simulink model "MTDC_MODEL"  (R2021a)
settings: Solver=ode1  StartTime=0.0  StopTime=3  FixedStep=2e-5  MaxStep=1e-5  RelTol=1e-5  EnableMultiTasking=on
InitFcn:
  | tau_iac=ts_G_iac/4;                                         %Current loop speed
  | wAC=1/tau_iac;                                              %Frequency
  | L1AC=wAC/s;                                                 %Open loop IMC (L) transfer function to obtain a first order after closing the loop
  | Kp_AC=wAC*(Lg_1+La_1/2);                                    %Proportional constant of the controller
  | Ki_AC=wAC*(Rg_1+Ra_1/2);                                    %Integral constant of the controller
  | C_IMC_AC=(Kp_AC*s+Ki_AC)/s;                                 %IMC designed PI controller transfer function
  | TAC=minreal((C_IMC_AC)*G_iac/(1+(C_IMC_AC)*G_iac));         %Closed loop transfer function
  | 
  | tau_Pac=ts_G_P/4;
  | D = TAC*U_ll1;
  | [C_pi,info] = pidtune(D,'PI',1/tau_Pac);
  | Ki_P = C_pi.Ki;
  | 
  | tau_Qac=ts_G_Q/4;
  | [C_piq,info] = pidtune(D,'PI',1/tau_Qac);
  | Ki_Q = C_piq.Ki;
  | 
  | 
  | tau_isum=ts_G_isum/4;                                        %Current loop speed
  | wsum=1/tau_isum;                                             %Frequency
  | L1AC=wsum/s;                                                 %Open loop IMC (L) transfer function to obtain a first order after closing the loop
  | Kp_sum=wsum*(2*La_1);                                        %Proportional constant of the controller
  | Ki_sum=wsum*(2*Ra_1);                                        %Integral constant of the controller
  | C_IMC_sum=(Kp_sum*s+Ki_sum)/s;                               %IMC designed PI controller transfer function
  | 
  | Kp_sum_PR = wc*(2*La_1);
  | Ki_sum_PR = wc*(2*Ra_1);
  | PR = (Kp_sum_PR*s^2 + 2*wc*(Kp_sum_PR+Ki_sum_PR)*s +Kp_sum_PR*w0^2)/(s^2+2*wc*s+w0^2);
  | 
  | 
  | %Energy reference for a converter arm (sum of all the submodule energies)
  | ArmEnergyRef=1/2*Carm*ArmVoltageRef^2;                      %Energy reference for a converter leg
  | LegEnergy=ArmEnergyRef*2;                                   %References for the controllers (DC side)
  | TotalEnergyRef=ArmEnergyRef*6;                              %Reference of the total energy of the converter
  | EnergyDiffabRef=0;                                          %Reference for the energy difference between legs a and b
  | EnergyDiffacRef=0;                                          %Reference for the energy difference between legs b and c
  | 
  | %References for the controllers (AC side)
  | EnergyDiffUpLowRefa=0;                                      %Reference for the energy difference upper and lower arms of phase a
  | EnergyDiffUpLowRefb=0;                                      %Reference for the energy difference upper and lower arms of phase b
  | EnergyDiffUpLowRefc=0;                                      %Reference for the energy difference upper and lower arms of phase c
  |                                                             %Controller design
  | Kpenergy=50;                                                %Proportional gain
  | Kienergy=20;                                                %Integral gain
  | 
  | Kpenergyt=50;                                               %Proportional gain
  | Kienergyt=20;                                               %Integral gain
  | 
  | Q=3;
  | wn=50*2*pi;                                                 %Frequency to eliminate 50 Hz
  | N_50 = tf([1 0 wn^2],[1 2*wn/Q wn^2]);                       %Notch filter 1 design
  | wn=100*2*pi;                                                %Frequency to eliminate 100 Hz
  | N_100 = tf([1 0 wn^2],[1 2*wn/Q wn^2]);                      %Notch filter 2 design
  | Notch=N_50*N_100;                                            %Combination of both notch filters
  | 
  | Ibasedc1= 1000e6/640e3;                 %Nominal current peak DC
  | IsaturationinnerDC1=1.1*Ibasedc1/3;  %Saturation of the DC inner current
  | IsaturationinnerAC1=0.45*Ibasedc1/3; %0.45  %Saturation of the inner current (why edu used 10% - FYI I changed it to 45%)
  | 
  | 
  | ... (+30 lines)
values from neighbouring files (symbols this model uses):
  ArmVoltageRef = 640e3    (= 640000)    [MMC_PARAMETERS.m]
  Cap = 9.5e-3    (= 0.0095)    [MMC_PARAMETERS.m]
  Carm = Cap/N    (= 2.375e-05)    [MMC_PARAMETERS.m]
  f_grid = 50    [MMC_PARAMETERS.m]
  La_1 = 0.15*Zbase_1/2/pi/50    (= 0.0488923985178)    [MMC_PARAMETERS.m]
  Lg_1 = 0.18*Zbase_1/2/pi/50    (= 0.0586708782214)    [MMC_PARAMETERS.m]
  N = 400    [MMC_PARAMETERS.m]
  Ra_1 = 0.01*Zbase_1    (= 1.024)    [MMC_PARAMETERS.m]
  Rg_1 = 0.005*Zbase_1    (= 0.512)    [MMC_PARAMETERS.m]
  S_1 = 1000e6    (= 1000000000)    [MMC_PARAMETERS.m]
  U_ll1 = 320e3    (= 320000)    [MMC_PARAMETERS.m]
  Vdc = 640e3    (= 640000)    [MMC_PARAMETERS.m]
  Vpeak_d1 = U_pnpeak1    [MMC_PARAMETERS.m]
  w0 = 2*pi*50    (= 314.159265359)    [MMC_PARAMETERS.m]
undefined symbols (not defined in the file or in its folder): Kp_Pac, lenght
libraries: spsSeriesRLCBranchLib x80, spsCurrentMeasurementLib x64, spsControlledVoltageSourceLib x36, pid_lib x32, spsVoltageMeasurementLib x32, spsControlledCurrentSourceLib x24, spsParallelRLCBranchLib x20, spsGroundLib x10, powerlib_extras x4, spsDCVoltageSourceLib x4, spspowerguiLib x1
(part 3 of 9)

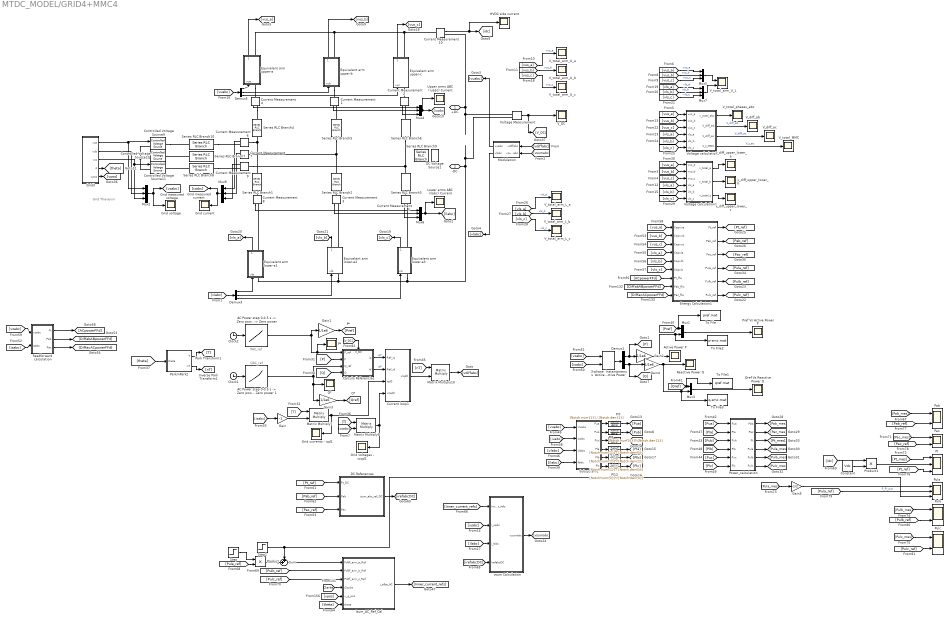
== system MTDC_MODEL/GRID4+MMC4 ==
  note: PAC_ref
  note: Grid Thevenin
  note: QAC_ref
  3-phase  Instantaneous  Active & Reactive Power : powerlib_extras/Measurements/3-phase  Instantaneous  Active & Reactive Power
      settings: SourceProductBaseCode=PS
  "AC Power step 0-0.5 s -> Zero power 0.5-2 s -> Active power injection 2 - 3 s -> Zero power " : Lookup_n-D  NumberOfTableDimensions=1  BreakpointsForDimension1=[0,0.5,2]  Table=[0,100e6,0]  InterpMethod=Flat  RndMeth=Simplest  InputSameDT=on
  "AC Power step 0-0.5 s -> Zero power 0.5-2 s -> Reactive power injection 2 - 3 s -> Zero power 1" : Lookup_n-D  NumberOfTableDimensions=1  BreakpointsForDimension1=[0,1,2]  Table=[0,5e6,0]  InterpMethod=Flat  RndMeth=Simplest  InputSameDT=on
  Active Power P : Scope
  Calculo Referencias : Subsystem
      settings: PortSchema="{\"entries\":[{\"content\":{\"sides\":[{\"content\":{\"connectorIds\":[\"In1\",\"In2\",\"In3\",\"In4\"]},\"type\":\"ConnectorPlacement.EquallySpacedRectSide\",\"uuid\":\"f5831c6a-58f5-4c55-8e24-523faf20dc0e\"},{\"content\":{\"connectorIds\":[\"Out1\",\"Out2\"],\"side\":\"RIGHT\"},\"type\":\"ConnectorPlacement.EquallySpacedRectSide\",\"uuid\":\"8e89a825-42f3-407f-8ce2-a529bb4d6e75\"},{\"content\":{\"connectorIds\":[\"In5\"],\"side\":\"TOP\"},\"type\":\"ConnectorPlacement.EquallySpacedRectSide\",\"uuid\":\"db0af466-562a-4a22-9801-d0efcc420c94\"},{\"content\":{\"connectorIds\":[],\"side\":\"BOTTOM\"},\"type\":\"ConnectorPlacement.EquallySpacedRectSide\",\"uuid\":\"e71aeab6-b02a-4177-93b6-e0e9fbfda2d5\"}]},\"type\":\"ConnectorPlacement.EquallySpacedConnector\",\"uuid\":\"54c33138-0c8b-4291-a3b0-05da54bcdffb\"}],\"packageUris\":[\"http://schema.mathworks.com/mf0/Connector/R2020b\"],\"version\":\"1.0\"}"
  Clock1 : Clock
  Clock2 : Clock
  Constant : Constant  Value=Vdc
  Controlled Voltage Source10 : spsControlledVoltageSourceLib/Controlled Voltage Source  Initialize=off  Source_Type=AC  Amplitude=0  Phase=0  Frequency=0  Measurements=None
  Controlled Voltage Source11 : spsControlledVoltageSourceLib/Controlled Voltage Source  Initialize=off  Source_Type=AC  Amplitude=0  Phase=0  Frequency=0  Measurements=None
  Controlled Voltage Source9 : spsControlledVoltageSourceLib/Controlled Voltage Source  Initialize=off  Source_Type=AC  Amplitude=0  Phase=0  Frequency=0  Measurements=None
  Current Measurement{1..10} (10 alike) : spsCurrentMeasurementLib/Current Measurement  PhasorSimulation=off  OutputType=Complex  PSBequivalent=0
  Current loop1 : Subsystem
  DC References : Subsystem
  DC Voltage Source1 : spsDCVoltageSourceLib/DC Voltage Source  Amplitude=Vdc  Measurements=None
  Demux1 : Demux  Outputs=2
  Demux3 : Demux  Outputs=3
  Demux5 : Demux  Outputs=3
  Energy Calculation1 : Subsystem
  Equivalent arm lower-a1 : Subsystem
  Equivalent arm lower-a2 : Subsystem
  Equivalent arm lower-a3 : Subsystem
  Equivalent arm upper-a : Subsystem
  Equivalent arm upper-b : Subsystem
  Equivalent arm upper-c : Subsystem
  Feedforward calculation : Subsystem
  Gain : Gain  Gain=-1
  Gain{1..4} (4 alike) : Gain  Gain=1/1e6
  Gain5 : Gain  Gain=-1/2
  Grid current : Scope
  Grid currents - iqd1 : Scope
  Grid voltage : Scope
  Grid voltages - vzqd1 : Scope
  Grid3 : Subsystem
  HVDC side current : Scope
  Isum_AC_Ref_Cal : Subsystem
  Lower arms ABC (ilabc) Current : Scope
  Matrix Multiply10 : Product  Multiplication=Matrix(*)
  Matrix Multiply5 : Product  Multiplication=Matrix(*)
  Matrix Multiply7 : Product  Multiplication=Matrix(*)
  Modulation : Subsystem
  Mux1 : Mux  Inputs=2
  Mux{2,4..7,9} (6 alike) : Mux  Inputs=3
  Mux3 : Mux  Inputs=2
  P* : Scope
  PI{7..12} (6 alike) : TransferFcn  Numerator=[Notch.num{1}]  Denominator=[Notch.den{1}]
  Pab : Scope  NumInputPorts=2
  Pac : Scope  NumInputPorts=2
  Park/nPark2 : Subsystem
  Power_calculation : Subsystem
  Pref Vs Active Power P : Scope
  Product : Product
  Product1 : Product
  Pt : Scope  NumInputPorts=3
  Pula : Scope  NumInputPorts=3
  Pulb : Scope  NumInputPorts=2
  Pulc : Scope  NumInputPorts=2
  Q* : Scope
  Qref Vs Reactive Power Q : Scope
  Reactive Power Q : Scope
  Series RLC Branch{1..6} (6 alike) : spsSeriesRLCBranchLib/Series RLC Branch  LConnTagsString=__new0  RConnTagsString=__new0  BranchType=RL  Resistance=Ra_1  Inductance=La_1  SetiL0=off  InitialCurrent=0  Capacitance=0  Setx0=off  InitialVoltage=0  Measurements=None
  Series RLC Branch10 : spsSeriesRLCBranchLib/Series RLC Branch  LConnTagsString=__new0  RConnTagsString=__new0  BranchType=RL  Resistance=Rg_1  Inductance=Lg_1  SetiL0=off  InitialCurrent=0  Capacitance=0  Setx0=off  InitialVoltage=0  Measurements=None
  Series RLC Branch7 : spsSeriesRLCBranchLib/Series RLC Branch  LConnTagsString=__new0  RConnTagsString=__new0  BranchType=RL  Resistance=Rg_1  Inductance=Lg_1  SetiL0=off  InitialCurrent=0  Capacitance=0  Setx0=off  InitialVoltage=0  Measurements=None
  Series RLC Branch8 : spsSeriesRLCBranchLib/Series RLC Branch  LConnTagsString=__new0  RConnTagsString=__new0  BranchType=RL  Resistance=Rg_1  Inductance=Lg_1  SetiL0=off  InitialCurrent=0  Capacitance=0  Setx0=off  InitialVoltage=0  Measurements=None
  Series RLC Branch9 : spsSeriesRLCBranchLib/Series RLC Branch  LConnTagsString=__new0  RConnTagsString=__new0  BranchType=C  Resistance=1  Inductance=1e-3  SetiL0=off  InitialCurrent=0  Capacitance=6*Carm  Setx0=off  InitialVoltage=0  Measurements=None
  Step : Step  Time=2.1  Before=1  After=0  SampleTime=0
  Step1 : Step  Time=2.1  After=-1e6  SampleTime=0
  Subsystem1 : Subsystem
  Sum : Sum  Inputs=++|
  To File : ToFile  Filename=pref.mat  MatrixName=ans0008  SaveFormat=Timeseries
  To File1 : ToFile  Filename=qref.mat  MatrixName=ans00010  SaveFormat=Timeseries
  To File2 : ToFile  Filename=p-smc.mat  MatrixName=ans0009  SaveFormat=Timeseries
  To File3 : ToFile  Filename=q-smc.mat  MatrixName=ans00011  SaveFormat=Timeseries
  Upper arms ABC (iuabc) Current : Scope
  V_DC : Scope
  V_diff_ab : Scope
  V_diff_ac : Scope
  V_total_MMC : Scope
  V_total_arm_L_a : Scope
  V_total_arm_L_b : Scope
  V_total_arm_L_c : Scope
  V_total_arm_U_L : Scope  NumInputPorts=2
  V_total_arm_U_a : Scope
  V_total_arm_U_b : Scope
  V_total_arm_U_c : Scope
  V_total_phases_abc : Scope
  Voltage Measurement : spsVoltageMeasurementLib/Voltage Measurement  PhasorSimulation=off  OutputType=Complex  PSBequivalent=0
  Voltage calculation : Subsystem
  Voltage calculation1 : Subsystem
  v_diff_upper_lower_a : Scope
  v_diff_upper_lower_b : Scope
  v_diff_upper_lower_c : Scope
  vsum Calculation : Subsystem
  +DC : PMIOPort  Side=Left
  -DC : PMIOPort  Port=2  Side=Left
  wires:
  [Inner_current_refs] -> vsum Calculation/1(Inner_current_refs)
  Current Measurement10/1 -> [idc], HVDC side current/1
  [Pla] -> Power_calculation/2(Pla)
  Grid3/4(thetareal) -> [theta]
  [Pulb_ref] -> Isum_AC_Ref_Cal/2(Pdiff_arm_b_Ref)
  Grid3/2(vzb) -> Mux2/2, Controlled Voltage Source10/1
  [vls_a] -> Energy Calculation1/4(Capvla)
  Demux3/1 -> Equivalent arm lower-a1/1(vla)
  Current Measurement5/1 -> Mux6/3
  Energy Calculation1/5(Pulb_ref) -> [Pulb_ref]
  Current Measurement8/1 -> Mux6/1
  Energy Calculation1/6(Pulc_ref) -> [Pulc_ref]
  Isum_AC_Ref_Cal/1(i_albe_AC) -> [Inner_current_refs]
  [Pt_ref] -> DC References/1(Pt_DC)
  3-phase  Instantaneous  Active & Reactive Power/1 -> Demux1/1
  Demux3/3 -> Equivalent arm lower-a3/1(vlc)
  [vls_c] -> Voltage calculation1/6(vls_c)
  Equivalent arm lower-a3/1(v_sum_lc) -> [vls_c]
  [Q] -> Calculo Referencias/4(Q)
  PI7/1 -> [Pua]
  Demux5/2 -> Equivalent arm upper-b/1(vub)
  Power_calculation/4(Pula) -> [Pula_mes]
  [vuabc] -> Subsystem1/1(Uuabc)
  [iuabc] -> Subsystem1/2(Iuabc)
  Current Measurement1/1 -> Mux4/2
  [vuabc] -> Demux5/1
  Current Measurement4/1 -> Mux4/1
  [vls_a] -> V_total_arm_L_a/1  "vls_a"
  Voltage calculation1/3(v_total_c) -> v_diff_upper_lower_c/1
  Energy Calculation1/1(Pt_ref) -> [Pt_ref]
  [vlabc] -> Demux3/1
  [Pulb_ref] -> Pulb/2
  [vus_b] -> Voltage calculation/2(vus_b)
  [Pt_mes] -> Pt/1
  [ilabc] -> Subsystem1/4(Ilabc)
  Current Measurement6/1 -> Mux9/1
  Demux1/2 -> Gain4/1, [Q]
  Voltage calculation/2(V_diff_ab) -> V_diff_ab/1  "V_diff_ab"
  Feedforward calculation/3(Pac) -> [DiffacACpowerFFd]
  Mux9/1 -> Grid current/1, [isabc]
  Feedforward calculation/1(Pt) -> [ACpowerFFd]
  [Clarke] -> Isum_AC_Ref_Cal/4(Clarke)
  [vzabc] -> Feedforward calculation/1(vzabc)
  [vls_b] -> Voltage calculation/5(vls_b)
  [theta] -> Isum_AC_Ref_Cal/6(theta)
  [vus_a] -> Voltage calculation/1(vus_a)
  [Pulc_ref] -> Isum_AC_Ref_Cal/3(Pdiff_arm_c_Ref)
  [isabc] -> Feedforward calculation/2(isabc)
  [DiffacACpowerFFd] -> Energy Calculation1/9(Pac_ffw)
  [iuabc] -> vsum Calculation/2(i_uabc)
  [ilabc] -> vsum Calculation/3(i_labc)
  Subsystem1/4(Pla) -> PI10/1
  Grid3/3(vzc) -> Mux2/3, Controlled Voltage Source11/1
  [Pab_mes] -> Pab/1
  Subsystem1/6(Plc) -> PI12/1
  Grid3/5(vpos) -> [vpos]
  Demux5/1 -> Equivalent arm upper-a/1(vua)
  [Pab_ref] -> Pab/2
  Matrix Multiply5/1 -> Current loop1/4(vzqd0), Grid voltages - vzqd1/1
  Subsystem1/5(Plb) -> PI11/1
  [vls_c] -> Mux7/3  "vls_c"
  [Pac_ref] -> Pac/2
  Mux4/1 -> [iuabc], Upper arms ABC (iuabc) Current/1
  Energy Calculation1/3(Pac_ref) -> [Pac_ref]
  Demux5/3 -> Equivalent arm upper-c/1(vuc)
  Power_calculation/1(Pab) -> [Pab_mes]
  [Pulc_mes] -> Pulc/1
  "AC Power step 0-0.5 s -> Zero power 0.5-2 s -> Active power injection 2 - 3 s -> Zero power "/1 -> Gain1/1, Calculo Referencias/1(P_ref), P*/1
  PI8/1 -> [Pub]
  Current Measurement7/1 -> Mux9/2
  [Plb] -> Power_calculation/4(Plb)
  [Pulc_ref] -> Pulc/2
  Mux5/1 -> V_total_arm_U_L/1
  Gain5/1 -> Pula/1
  Power_calculation/6(Pulc) -> [Pulc_mes]
  PI10/1 -> [Pla]
  Energy Calculation1/4(Pula_ref) -> [Pula_ref]
  [vzabc] -> Matrix Multiply5/2
  Gain4/1 -> Reactive Power Q/1, To File3/1, Mux3/2
  PI9/1 -> [Puc]
  [Pulb_mes] -> Pulb/1
  [Pref] -> To File/1, Mux1/1
  [vus_c] -> Voltage calculation1/3(vus_c)
  [Pt_ref] -> Pt/3
  Power_calculation/5(Pulb) -> [Pulb_mes]
  [Pab_ref] -> DC References/2(Pab)
  Sum/1 -> Isum_AC_Ref_Cal/1(Pdiff_arm_a_Ref)
  [vus_a] -> V_total_arm_U_a/1  "vus_a"
  Voltage calculation/1(v_total_abc) -> V_total_phases_abc/1
  Modulation/1(vuabc) -> [vuabc]
  Product/1 -> Sum/2
  Mux7/1 -> V_total_arm_U_L/2
  Calculo Referencias/1(iq) -> Current loop1/1(Ref_iq)  "iq*"
  [Puc] -> Power_calculation/5(Puc)
  PI12/1 -> [Plc]
  Power_calculation/2(Pac) -> [Pac_mes]
  vsum Calculation/1(vsumabc) -> [vsumabc]
  [vsumabc] -> Modulation/2(vsumabc)
  Voltage Measurement/1 -> V_DC/1, [V_DC]
  Feedforward calculation/2(Pab) -> [DiffabABpowerFFd]
  [T] -> Matrix Multiply7/1
  [Pac_mes] -> Pac/1
  [Pub] -> Power_calculation/3(Pub)
  Step/1 -> Product/1
  Demux1/1 -> Gain2/1, [P]
  [Pac_ref] -> DC References/3(Pac)
  DC References/1(isum_abc_ref_DC) -> [irefabcDC]
  PI11/1 -> [Plb]
  Mux1/1 -> Pref Vs Active Power P/1
  [Pula_mes] -> Gain5/1
  [vus_a] -> Voltage calculation1/1(vus_a)
  [irefabcDC] -> vsum Calculation/4(irefabcDC)
  [vls_c] -> Energy Calculation1/6(Capvlc)
  [Pula_ref] -> Pula/2  "P_PI_out"
  Subsystem1/1(Pua) -> PI7/1
  [vus_c] -> Energy Calculation1/3(Capvuc)
  [vls_a] -> Voltage calculation1/4(vls_a)
  [DiffabABpowerFFd] -> Energy Calculation1/8(Pab_ffw)
  Power_calculation/3(Pt) -> [Pt_mes]
  [idc] -> Product1/1
  [ACpowerFFd] -> Energy Calculation1/7(Pt_ffw)
  Product1/1 -> Pt/2
  Step1/1 -> Sum/1, Pula/3
  [Pula_ref] -> Product/2
  [vpos] -> Isum_AC_Ref_Cal/5(v_g_pos)
  Gain/1 -> Matrix Multiply7/2
  [vus_a] -> Mux5/1  "vus_a"
  [vlabc] -> Subsystem1/3(Ulabc)
  Clock1/1 -> "AC Power step 0-0.5 s -> Zero power 0.5-2 s -> Reactive power injection 2 - 3 s -> Zero power 1"/1
  Matrix Multiply7/1 -> Grid currents - iqd1/1, Current loop1/3(iqd0)
  Clock2/1 -> "AC Power step 0-0.5 s -> Zero power 0.5-2 s -> Active power injection 2 - 3 s -> Zero power "/1
  Demux3/2 -> Equivalent arm lower-a2/1(vlb)
  Constant/1 -> Product1/2
  [vls_b] -> Voltage calculation1/5(vls_b)
  [vus_b] -> Voltage calculation1/2(vus_b)
  [vls_c] -> Voltage calculation/6(vls_c)
  Voltage calculation1/1(v_total_a) -> v_diff_upper_lower_a/1
  [vls_a] -> Mux7/1  "vls_a"
  [vls_b] -> Mux7/2  "vls_b"
  Equivalent arm upper-b/1(v_sum_ub) -> [vus_b]
  [vls_b] -> V_total_arm_L_b/1  "vls_b"
  [isabc] -> Gain/1
  [vus_c] -> Voltage calculation/3(vus_c)
  [vus_b] -> Mux5/2  "vus_b"
  Mux3/1 -> Qref Vs Reactive Power Q/1
  [vus_b] -> V_total_arm_U_b/1  "vus_b"
  Voltage calculation/3(V_diff_ac) -> V_diff_ac/1  "V_diff_ac"
  [vus_c] -> Mux5/3  "vus_c"
  [vus_c] -> V_total_arm_U_c/1  "vus_c"
  Equivalent arm lower-a1/1(v_sum_la) -> [vls_a]
  "AC Power step 0-0.5 s -> Zero power 0.5-2 s -> Reactive power injection 2 - 3 s -> Zero power 1"/1 -> Q*/1, Gain3/1, Calculo Referencias/3(Q_ref)
  Equivalent arm lower-a2/1(v_sum_lb) -> [vls_b]
  Mux2/1 -> Grid voltage/1, [vzabc]
  Current loop1/1(vlqd0) -> Matrix Multiply10/2
  Grid3/1(vza) -> Mux2/1, Controlled Voltage Source9/1
  Gain2/1 -> Active Power P/1, To File2/1, Mux1/2
  [Qref] -> To File1/1, Mux3/1
  Voltage calculation/4(V_t_MMC) -> V_total_MMC/1  "V_t_ac"
  Park/nPark2/1(T) -> [T]
  Calculo Referencias/2(id) -> Current loop1/2(Ref_id)  "id*"
  [T] -> Matrix Multiply5/1
  Modulation/2(vlabc) -> [vlabc]
  Gain3/1 -> [Qref]
  Equivalent arm upper-c/1(v_sum_uc) -> [vus_c]
  [nT] -> Matrix Multiply10/1
  Park/nPark2/2("nT ") -> [nT]
  [P] -> Calculo Referencias/2(P)
  [vls_a] -> Voltage calculation/4(vls_a)
  [theta] -> Park/nPark2/1(theta)
  Mux6/1 -> [ilabc], Lower arms ABC (ilabc) Current/1
  Matrix Multiply10/1 -> [vdiffabc]
  [isabc] -> 3-phase  Instantaneous  Active & Reactive Power/2
  [Plc] -> Power_calculation/6(Plc)
  Equivalent arm upper-a/1(v_sum_ua) -> [vus_a]
  Current Measurement2/1 -> Mux4/3
  [vzabc] -> 3-phase  Instantaneous  Active & Reactive Power/1
  [vdiffabc] -> Modulation/1(vdiffabc)
  [Pua] -> Power_calculation/1(Pua)
  Subsystem1/3(Puc) -> PI9/1
  [vls_c] -> V_total_arm_L_c/1  "vls_c"
  Current Measurement9/1 -> Mux9/3
  Gain1/1 -> [Pref]
  [vls_b] -> Energy Calculation1/5(Capvlb)
  Subsystem1/2(Pub) -> PI8/1
  [vus_a] -> Energy Calculation1/1(Capvua)
  Voltage calculation1/2(v_total_b) -> v_diff_upper_lower_b/1
  Energy Calculation1/2(Pab_ref) -> [Pab_ref]
  [vus_b] -> Energy Calculation1/2(Capvub)
  Current Measurement3/1 -> Mux6/2
  [V_DC] -> Calculo Referencias/5(V_DC)
  connections:
  Equivalent arm upper-b/LConn1 -- Current Measurement1/LConn1
  Equivalent arm upper-a/LConn1 -- Current Measurement4/LConn1
  Controlled Voltage Source9/RConn1 -- Series RLC Branch10/LConn1
  Series RLC Branch5/LConn1 -- Current Measurement1/RConn1
  Equivalent arm lower-a2/RConn1 -- Current Measurement3/RConn1
  Series RLC Branch6/LConn1 -- Current Measurement2/RConn1
  Equivalent arm upper-c/LConn1 -- Current Measurement2/LConn1
  Series RLC Branch2/RConn1 -- Current Measurement3/LConn1
  Series RLC Branch1/RConn1 -- Current Measurement8/LConn1
  Series RLC Branch7/RConn1 -- Current Measurement7/RConn1
  Series RLC Branch8/LConn1 -- Controlled Voltage Source11/RConn1
  Series RLC Branch3/RConn1 -- Current Measurement5/LConn1
  Equivalent arm lower-a3/RConn1 -- Current Measurement5/RConn1
  Equivalent arm lower-a1/RConn1 -- Current Measurement8/RConn1
  Series RLC Branch7/LConn1 -- Controlled Voltage Source10/RConn1
  Series RLC Branch10/RConn1 -- Current Measurement6/RConn1
  Current Measurement4/RConn1 -- Series RLC Branch4/LConn1
  Series RLC Branch8/RConn1 -- Current Measurement9/RConn1
  Series RLC Branch3/LConn1 -- Series RLC Branch6/RConn1 -- Current Measurement9/LConn1
  Series RLC Branch2/LConn1 -- Series RLC Branch5/RConn1 -- Current Measurement7/LConn1
  Equivalent arm upper-b/RConn1 -- Equivalent arm upper-c/RConn1 -- Current Measurement10/LConn1 -- Equivalent arm upper-a/RConn1
  Controlled Voltage Source11/LConn1 -- Controlled Voltage Source9/LConn1 -- Controlled Voltage Source10/LConn1
  +DC/RConn1 -- Current Measurement10/RConn1 -- Voltage Measurement/LConn1
  Series RLC Branch1/LConn1 -- Series RLC Branch4/RConn1 -- Current Measurement6/LConn1
  Equivalent arm lower-a3/LConn1 -- -DC/RConn1 -- Voltage Measurement/LConn2 -- Equivalent arm lower-a2/LConn1 -- Equivalent arm lower-a1/LConn1

== system MTDC_MODEL/GRID1+MMC1/Calculo Referencias ==
  P_ref : Inport
  P : Inport  Port=2
  Q_ref : Inport  Port=3
  Q : Inport  Port=4
  V_DC : Inport  Port=5
  Constant : Constant  Value=Vdc*1.00
  Constant1 : Constant  Value=sqrt(2)*1000*Vdc/(3*U_ll1)
  Gain : Gain  Gain=-1
  Gain1 : Gain  Gain=-1
  Gain2 : Gain
  PID Controller1 : pid_lib/PID Controller  Controller=I  Form=Parallel  TimeDomain=Continuous-time  UseExternalTs=off  SampleTime=1  IntegratorMethod=Forward Euler  FilterMethod=Forward Euler  ControllerParametersSource=internal  P=Kp_Pac  I=Ki_Q  D=0  UseFilter=on  N=100  TunerSelectOption=Transfer Function Based (PID Tuner App)  InitialConditionSource=internal  InitialConditionForIntegrator=0  InitialConditionForFilter=0  DifferentiatorICPrevScaledInput=0  ExternalReset=none  TrackingMode=off  Kt=1  LimitOutput=off  SatLimitsSource=internal  UpperSaturationLimit=inf  LowerSaturationLimit=-inf  LinearizeAsGain=on  AntiWindupMode=none  Kb=1  POutMin=[]  POutMax=[]  IOutMin=[]  IOutMax=[]  DOutMin=[]  DOutMax=[]  NOutMin=[]  NOutMax=[]  SumOutMin=[]  SumOutMax=[]  SaturationOutMin=[]  SaturationOutMax=[]  PParamMin=[]  PParamMax=[]  IParamMin=[]  IParamMax=[]  DParamMin=[]  DParamMax=[]  NParamMin=[]  NParamMax=[]  KbParamMin=[]  KbParamMax=[]  KtParamMin=[]  KtParamMax=[]  KbOutMin=[]  KbOutMax=[]  KtOutMin=[]  KtOutMax=[]  IntegratorOutMin=[]  IntegratorOutMax=[]  FilterOutMin=[]  FilterOutMax=[]  SumI1OutMin=[]  SumI1OutMax=[]  SumI2OutMin=[]  SumI2OutMax=[]  SumI3OutMin=[]  SumI3OutMax=[]  SumI4OutMin=[]  SumI4OutMax=[]  SumDOutMin=[]  SumDOutMax=[]  DifferentiatorOutMin=[]  DifferentiatorOutMax=[]  FilterDiffOutCoefMin=[]  FilterDiffOutCoefMax=[]  ReciprocalOutMin=[]  ReciprocalOutMax=[]  SumDenOutMin=[]  SumDenOutMax=[]  SumNumOutMin=[]  SumNumOutMax=[]  DivideOutMin=[]  DivideOutMax=[]  UdiffTsProdOutMin=[]  UdiffTsProdOutMax=[]  NTsProdOutMin=[]  NTsProdOutMax=[]  UintegralTsProdOutMin=[]  UintegralTsProdOutMax=[]  UngainTsProdOutMin=[]  UngainTsProdOutMax=[]  IntegratorContinuousStateAttributes=''  IntegratorStateMustResolveToSignalObject=off  IntegratorRTWStateStorageClass=Auto  FilterContinuousStateAttributes=''  FilterStateMustResolveToSignalObject=off  FilterRTWStateStorageClass=Auto  ParallelPVariant=Disabled  IdealPVariant=Disabled  IVariant=InternalParameters  DVariant=Disabled  IntegratorVariant=Continuous  SatVariant=Disabled  AWVariant=Passthrough  PCopyVariant=Disabled  TRVariant=Disabled  FdbkBlocksVariant=Forward  IdealPFdbkVariant=Disabled  SatFdbkVariant=Disabled  DerivativeFilterVariant=Disabled  NVariant=Disabled  NCopyVariant=Disabled_SignalSpec  FilterICVariant=Disabled  IntegratorICVariant=InternalICs  ExternalResetVariant=Disabled  TRSumVariant=Passthrough  SumFdbkVariant=Disabled  SumVariant=Passthrough_I  TsampFilterVariant=InternalTs  TsampNgainVariant=Passthrough  TsampIntegralVariant=Passthrough  ExternalSaturationOutDataTypeStr=Inherit: Same as second input
  PID Controller2 : pid_lib/PID Controller  Controller=PI  Form=Parallel  TimeDomain=Continuous-time  UseExternalTs=off  SampleTime=1  IntegratorMethod=Forward Euler  FilterMethod=Forward Euler  ControllerParametersSource=internal  P=3e-5  I=77e-4  D=0  UseFilter=on  N=100  TunerSelectOption=Transfer Function Based (PID Tuner App)  ZeroCross=off  InitialConditionSource=internal  InitialConditionForIntegrator=0  InitialConditionForFilter=0  DifferentiatorICPrevScaledInput=0  ExternalReset=none  TrackingMode=off  Kt=1  LimitOutput=off  SatLimitsSource=internal  UpperSaturationLimit=inf  LowerSaturationLimit=-inf  LinearizeAsGain=on  AntiWindupMode=none  Kb=1  POutMin=[]  POutMax=[]  IOutMin=[]  IOutMax=[]  DOutMin=[]  DOutMax=[]  NOutMin=[]  NOutMax=[]  SumOutMin=[]  SumOutMax=[]  SaturationOutMin=[]  SaturationOutMax=[]  PParamMin=[]  PParamMax=[]  IParamMin=[]  IParamMax=[]  DParamMin=[]  DParamMax=[]  NParamMin=[]  NParamMax=[]  KbParamMin=[]  KbParamMax=[]  KtParamMin=[]  KtParamMax=[]  KbOutMin=[]  KbOutMax=[]  KtOutMin=[]  KtOutMax=[]  IntegratorOutMin=[]  IntegratorOutMax=[]  FilterOutMin=[]  FilterOutMax=[]  SumI1OutMin=[]  SumI1OutMax=[]  SumI2OutMin=[]  SumI2OutMax=[]  SumI3OutMin=[]  SumI3OutMax=[]  SumI4OutMin=[]  SumI4OutMax=[]  SumDOutMin=[]  SumDOutMax=[]  DifferentiatorOutMin=[]  DifferentiatorOutMax=[]  FilterDiffOutCoefMin=[]  FilterDiffOutCoefMax=[]  ReciprocalOutMin=[]  ReciprocalOutMax=[]  SumDenOutMin=[]  SumDenOutMax=[]  SumNumOutMin=[]  SumNumOutMax=[]  DivideOutMin=[]  DivideOutMax=[]  UdiffTsProdOutMin=[]  UdiffTsProdOutMax=[]  NTsProdOutMin=[]  NTsProdOutMax=[]  UintegralTsProdOutMin=[]  UintegralTsProdOutMax=[]  UngainTsProdOutMin=[]  UngainTsProdOutMax=[]  IntegratorContinuousStateAttributes=''  IntegratorStateMustResolveToSignalObject=off  IntegratorRTWStateStorageClass=Auto  FilterContinuousStateAttributes=''  FilterStateMustResolveToSignalObject=off  FilterRTWStateStorageClass=Auto  ParallelPVariant=InternalParameters  IdealPVariant=Disabled  IVariant=InternalParameters  DVariant=Disabled  IntegratorVariant=Continuous  SatVariant=Disabled  AWVariant=Passthrough  PCopyVariant=Disabled  TRVariant=Disabled  FdbkBlocksVariant=Forward  IdealPFdbkVariant=Disabled  SatFdbkVariant=Disabled  DerivativeFilterVariant=Disabled  NVariant=Disabled  NCopyVariant=Disabled_SignalSpec  FilterICVariant=Disabled  IntegratorICVariant=InternalICs  ExternalResetVariant=Disabled  TRSumVariant=Passthrough  SumFdbkVariant=Disabled  SumVariant=Sum_PI  TsampFilterVariant=InternalTs  TsampNgainVariant=Passthrough  TsampIntegralVariant=Passthrough  ExternalSaturationOutDataTypeStr=Inherit: Same as second input
  PID Controller4 : pid_lib/PID Controller  Controller=I  Form=Parallel  TimeDomain=Continuous-time  UseExternalTs=off  SampleTime=1  IntegratorMethod=Forward Euler  FilterMethod=Forward Euler  ControllerParametersSource=internal  P=Kp_Pac  I=Ki_P  D=0  UseFilter=on  N=100  TunerSelectOption=Transfer Function Based (PID Tuner App)  InitialConditionSource=internal  InitialConditionForIntegrator=0  InitialConditionForFilter=0  DifferentiatorICPrevScaledInput=0  ExternalReset=none  TrackingMode=off  Kt=1  LimitOutput=off  SatLimitsSource=internal  UpperSaturationLimit=inf  LowerSaturationLimit=-inf  LinearizeAsGain=on  AntiWindupMode=none  Kb=1  POutMin=[]  POutMax=[]  IOutMin=[]  IOutMax=[]  DOutMin=[]  DOutMax=[]  NOutMin=[]  NOutMax=[]  SumOutMin=[]  SumOutMax=[]  SaturationOutMin=[]  SaturationOutMax=[]  PParamMin=[]  PParamMax=[]  IParamMin=[]  IParamMax=[]  DParamMin=[]  DParamMax=[]  NParamMin=[]  NParamMax=[]  KbParamMin=[]  KbParamMax=[]  KtParamMin=[]  KtParamMax=[]  KbOutMin=[]  KbOutMax=[]  KtOutMin=[]  KtOutMax=[]  IntegratorOutMin=[]  IntegratorOutMax=[]  FilterOutMin=[]  FilterOutMax=[]  SumI1OutMin=[]  SumI1OutMax=[]  SumI2OutMin=[]  SumI2OutMax=[]  SumI3OutMin=[]  SumI3OutMax=[]  SumI4OutMin=[]  SumI4OutMax=[]  SumDOutMin=[]  SumDOutMax=[]  DifferentiatorOutMin=[]  DifferentiatorOutMax=[]  FilterDiffOutCoefMin=[]  FilterDiffOutCoefMax=[]  ReciprocalOutMin=[]  ReciprocalOutMax=[]  SumDenOutMin=[]  SumDenOutMax=[]  SumNumOutMin=[]  SumNumOutMax=[]  DivideOutMin=[]  DivideOutMax=[]  UdiffTsProdOutMin=[]  UdiffTsProdOutMax=[]  NTsProdOutMin=[]  NTsProdOutMax=[]  UintegralTsProdOutMin=[]  UintegralTsProdOutMax=[]  UngainTsProdOutMin=[]  UngainTsProdOutMax=[]  IntegratorContinuousStateAttributes=''  IntegratorStateMustResolveToSignalObject=off  IntegratorRTWStateStorageClass=Auto  FilterContinuousStateAttributes=''  FilterStateMustResolveToSignalObject=off  FilterRTWStateStorageClass=Auto  ParallelPVariant=Disabled  IdealPVariant=Disabled  IVariant=InternalParameters  DVariant=Disabled  IntegratorVariant=Continuous  SatVariant=Disabled  AWVariant=Passthrough  PCopyVariant=Disabled  TRVariant=Disabled  FdbkBlocksVariant=Forward  IdealPFdbkVariant=Disabled  SatFdbkVariant=Disabled  DerivativeFilterVariant=Disabled  NVariant=Disabled  NCopyVariant=Disabled_SignalSpec  FilterICVariant=Disabled  IntegratorICVariant=InternalICs  ExternalResetVariant=Disabled  TRSumVariant=Passthrough  SumFdbkVariant=Disabled  SumVariant=Passthrough_I  TsampFilterVariant=InternalTs  TsampNgainVariant=Passthrough  TsampIntegralVariant=Passthrough  ExternalSaturationOutDataTypeStr=Inherit: Same as second input
  Product2 : Product
  Sum1 : Sum  Inputs=|+-
  Sum2 : Sum  Inputs=|+-
  Sum5 : Sum  Inputs=|+-
  i* : Scope  NumInputPorts=2
  i*1 : Scope  NumInputPorts=2
  iq : Outport
  id : Outport  Port=2
  wires:
  P_ref/1 -> Sum5/1
  P/1 -> Sum5/2
  Sum5/1 -> PID Controller4/1
  PID Controller4/1 -> Gain/1
  Sum1/1 -> PID Controller1/1
  Q_ref/1 -> Sum1/1
  Q/1 -> Sum1/2
  PID Controller1/1 -> Gain1/1
  Gain/1 -> i*/1
  Gain1/1 -> id/1, i*/2
  V_DC/1 -> Sum2/2
  Constant/1 -> Sum2/1
  Sum2/1 -> PID Controller2/1
  PID Controller2/1 -> Product2/1, i*1/2
  Gain2/1 -> iq/1, i*1/1
  Product2/1 -> Gain2/1
  Constant1/1 -> Product2/2

== system MTDC_MODEL/GRID1+MMC1/Current loop1 ==
  note: Grid voltage qd frame
  Ref_iq : Inport
  Ref_id : Inport  Port=2
  iqd0 : Inport  Port=3
  vzqd0 : Inport  Port=4
  Constant2 : Constant  Value=2*pi*50  SampleTime=-1
  Constant3 : Constant  Value=0
  Current control d axis PI Controller : pid_lib/PID Controller  Controller=PI  Form=Parallel  TimeDomain=Continuous-time  UseExternalTs=off  SampleTime=1  IntegratorMethod=Forward Euler  FilterMethod=Forward Euler  ControllerParametersSource=internal  P=Kp_AC  I=Ki_AC  D=0  UseFilter=on  N=100  TunerSelectOption=Transfer Function Based (PID Tuner App)  InitialConditionSource=internal  InitialConditionForIntegrator=0  InitialConditionForFilter=0  DifferentiatorICPrevScaledInput=0  ExternalReset=none  TrackingMode=off  Kt=1  LimitOutput=off  SatLimitsSource=internal  UpperSaturationLimit=inf  LowerSaturationLimit=-inf  LinearizeAsGain=on  AntiWindupMode=none  Kb=1  POutMin=[]  POutMax=[]  IOutMin=[]  IOutMax=[]  DOutMin=[]  DOutMax=[]  NOutMin=[]  NOutMax=[]  SumOutMin=[]  SumOutMax=[]  SaturationOutMin=[]  SaturationOutMax=[]  PParamMin=[]  PParamMax=[]  IParamMin=[]  IParamMax=[]  DParamMin=[]  DParamMax=[]  NParamMin=[]  NParamMax=[]  KbParamMin=[]  KbParamMax=[]  KtParamMin=[]  KtParamMax=[]  KbOutMin=[]  KbOutMax=[]  KtOutMin=[]  KtOutMax=[]  IntegratorOutMin=[]  IntegratorOutMax=[]  FilterOutMin=[]  FilterOutMax=[]  SumI1OutMin=[]  SumI1OutMax=[]  SumI2OutMin=[]  SumI2OutMax=[]  SumI3OutMin=[]  SumI3OutMax=[]  SumI4OutMin=[]  SumI4OutMax=[]  SumDOutMin=[]  SumDOutMax=[]  DifferentiatorOutMin=[]  DifferentiatorOutMax=[]  FilterDiffOutCoefMin=[]  FilterDiffOutCoefMax=[]  ReciprocalOutMin=[]  ReciprocalOutMax=[]  SumDenOutMin=[]  SumDenOutMax=[]  SumNumOutMin=[]  SumNumOutMax=[]  DivideOutMin=[]  DivideOutMax=[]  UdiffTsProdOutMin=[]  UdiffTsProdOutMax=[]  NTsProdOutMin=[]  NTsProdOutMax=[]  UintegralTsProdOutMin=[]  UintegralTsProdOutMax=[]  UngainTsProdOutMin=[]  UngainTsProdOutMax=[]  IntegratorContinuousStateAttributes=''  IntegratorStateMustResolveToSignalObject=off  IntegratorRTWStateStorageClass=Auto  FilterContinuousStateAttributes=''  FilterStateMustResolveToSignalObject=off  FilterRTWStateStorageClass=Auto  ParallelPVariant=InternalParameters  IdealPVariant=Disabled  IVariant=InternalParameters  DVariant=Disabled  IntegratorVariant=Continuous  SatVariant=Disabled  AWVariant=Passthrough  PCopyVariant=Disabled  TRVariant=Disabled  FdbkBlocksVariant=Forward  IdealPFdbkVariant=Disabled  SatFdbkVariant=Disabled  DerivativeFilterVariant=Disabled  NVariant=Disabled  NCopyVariant=Disabled_SignalSpec  FilterICVariant=Disabled  IntegratorICVariant=InternalICs  ExternalResetVariant=Disabled  TRSumVariant=Passthrough  SumFdbkVariant=Disabled  SumVariant=Sum_PI  TsampFilterVariant=InternalTs  TsampNgainVariant=Passthrough  TsampIntegralVariant=Passthrough  ExternalSaturationOutDataTypeStr=Inherit: Same as second input
  Current control q axis PI Controller : pid_lib/PID Controller  Controller=PI  Form=Parallel  TimeDomain=Continuous-time  UseExternalTs=off  SampleTime=1  IntegratorMethod=Forward Euler  FilterMethod=Forward Euler  ControllerParametersSource=internal  P=Kp_AC  I=Ki_AC  D=0  UseFilter=on  N=100  TunerSelectOption=Transfer Function Based (PID Tuner App)  InitialConditionSource=internal  InitialConditionForIntegrator=0  InitialConditionForFilter=0  DifferentiatorICPrevScaledInput=0  ExternalReset=none  TrackingMode=off  Kt=1  LimitOutput=off  SatLimitsSource=internal  UpperSaturationLimit=inf  LowerSaturationLimit=-inf  LinearizeAsGain=on  AntiWindupMode=none  Kb=1  POutMin=[]  POutMax=[]  IOutMin=[]  IOutMax=[]  DOutMin=[]  DOutMax=[]  NOutMin=[]  NOutMax=[]  SumOutMin=[]  SumOutMax=[]  SaturationOutMin=[]  SaturationOutMax=[]  PParamMin=[]  PParamMax=[]  IParamMin=[]  IParamMax=[]  DParamMin=[]  DParamMax=[]  NParamMin=[]  NParamMax=[]  KbParamMin=[]  KbParamMax=[]  KtParamMin=[]  KtParamMax=[]  KbOutMin=[]  KbOutMax=[]  KtOutMin=[]  KtOutMax=[]  IntegratorOutMin=[]  IntegratorOutMax=[]  FilterOutMin=[]  FilterOutMax=[]  SumI1OutMin=[]  SumI1OutMax=[]  SumI2OutMin=[]  SumI2OutMax=[]  SumI3OutMin=[]  SumI3OutMax=[]  SumI4OutMin=[]  SumI4OutMax=[]  SumDOutMin=[]  SumDOutMax=[]  DifferentiatorOutMin=[]  DifferentiatorOutMax=[]  FilterDiffOutCoefMin=[]  FilterDiffOutCoefMax=[]  ReciprocalOutMin=[]  ReciprocalOutMax=[]  SumDenOutMin=[]  SumDenOutMax=[]  SumNumOutMin=[]  SumNumOutMax=[]  DivideOutMin=[]  DivideOutMax=[]  UdiffTsProdOutMin=[]  UdiffTsProdOutMax=[]  NTsProdOutMin=[]  NTsProdOutMax=[]  UintegralTsProdOutMin=[]  UintegralTsProdOutMax=[]  UngainTsProdOutMin=[]  UngainTsProdOutMax=[]  IntegratorContinuousStateAttributes=''  IntegratorStateMustResolveToSignalObject=off  IntegratorRTWStateStorageClass=Auto  FilterContinuousStateAttributes=''  FilterStateMustResolveToSignalObject=off  FilterRTWStateStorageClass=Auto  ParallelPVariant=InternalParameters  IdealPVariant=Disabled  IVariant=InternalParameters  DVariant=Disabled  IntegratorVariant=Continuous  SatVariant=Disabled  AWVariant=Passthrough  PCopyVariant=Disabled  TRVariant=Disabled  FdbkBlocksVariant=Forward  IdealPFdbkVariant=Disabled  SatFdbkVariant=Disabled  DerivativeFilterVariant=Disabled  NVariant=Disabled  NCopyVariant=Disabled_SignalSpec  FilterICVariant=Disabled  IntegratorICVariant=InternalICs  ExternalResetVariant=Disabled  TRSumVariant=Passthrough  SumFdbkVariant=Disabled  SumVariant=Sum_PI  TsampFilterVariant=InternalTs  TsampNgainVariant=Passthrough  TsampIntegralVariant=Passthrough  ExternalSaturationOutDataTypeStr=Inherit: Same as second input
  Demux2 : Demux  Outputs=2
  Divide : Product  Inputs=**
  Divide1 : Product  Inputs=**
  Gain1 : Gain  Gain=(Lg_1+La_1/2)
  Mux1 : Mux  Inputs=2
  Mux3 : Mux  Inputs=2
  Mux5 : Mux  Inputs=2
  Scope1 : Scope
  Scope2 : Scope
  Scope7 : Scope
  Sum3 : Sum  Inputs=-+|
  Sum4 : Sum  Inputs=|++
  Sum5 : Sum  Inputs=|+-
  Sum7 : Sum  Inputs=|+-
  Sum8 : Sum  Inputs=--|
  iqd0-iqd : Selector  InputPortWidth=3  IndexOptions=Index vector (dialog)  Indices=[1 2]  OutputSizes=1
  vzqd0-vzqd : Selector  InputPortWidth=3  IndexOptions=Index vector (dialog)  Indices=[1 2]  OutputSizes=1
  vlqd0 : Outport
  wires:
  Ref_iq/1 -> Sum5/1
  Ref_id/1 -> Sum3/2
  Current control q axis PI Controller/1 -> Sum8/1
  Mux3/1 -> Sum4/1
  vzqd0-vzqd/1 -> Scope7/1, Sum4/2  "vzqd"
  Sum5/1 -> [error_iq], Current control q axis PI Controller/1
  Gain1/1 -> Divide1/1, Divide/2
  Constant2/1 -> Gain1/1
  Demux2/1 -> Divide1/2, Sum5/2
  Divide/1 -> Sum8/2
  vzqd0/1 -> vzqd0-vzqd/1  "vzqd0"
  Sum4/1 -> Mux5/1
  Sum7/1 -> Mux3/2
  Sum3/1 -> [error_id], Current control d axis PI Controller/1
  Divide1/1 -> Sum7/1
  Sum8/1 -> Mux3/1
  Current control d axis PI Controller/1 -> Sum7/2
  Constant3/1 -> Mux5/2
  Demux2/2 -> Sum3/1, Divide/1
  iqd0/1 -> iqd0-iqd/1
  iqd0-iqd/1 -> Demux2/1
  Mux5/1 -> Scope2/1, vlqd0/1
  [error_id] -> Mux1/2
  [error_iq] -> Mux1/1
  Mux1/1 -> Scope1/1

== system MTDC_MODEL/GRID1+MMC1/DC References ==
  Pt_DC : Inport
  Pab : Inport  Port=2
  Pac : Inport  Port=3
  Constant : Constant  Value=[1,1,1;1,-2,1;1,1,-2]
  Gain1 : Gain  Gain=1/(3*Vdc)
  Matrix Multiply2 : Product  Multiplication=Matrix(*)
  Mux10 : Mux  Inputs=3
  Sat3 : Subsystem
  isum_abc_ref_DC : Outport
  wires:
  Matrix Multiply2/1 -> Gain1/1
  Constant/1 -> Matrix Multiply2/1
  Mux10/1 -> Matrix Multiply2/2
  Gain1/1 -> Sat3/1(In1)  "isum_abc_ref_DC"
  Pt_DC/1 -> Mux10/1
  Pac/1 -> Mux10/3
  Pab/1 -> Mux10/2
  Sat3/1(Out1) -> isum_abc_ref_DC/1

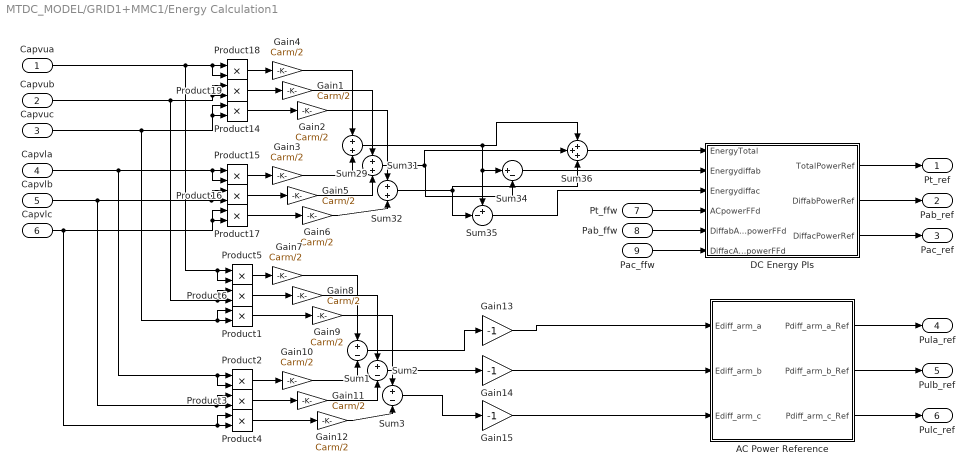
== system MTDC_MODEL/GRID1+MMC1/Energy Calculation1 ==
  Capvua : Inport
  Capvub : Inport  Port=2
  Capvuc : Inport  Port=3
  Capvla : Inport  Port=4
  Capvlb : Inport  Port=5
  Capvlc : Inport  Port=6
  Pt_ffw : Inport  Port=7
  Pab_ffw : Inport  Port=8
  Pac_ffw : Inport  Port=9
  AC Power Reference : Subsystem
  DC Energy PIs : Subsystem
  Gain{1..12} (12 alike) : Gain  Gain=Carm/2
  Gain13 : Gain  Gain=-1
  Gain14 : Gain  Gain=-1
  Gain15 : Gain  Gain=-1
  Product{1..6,14..19} (12 alike) : Product
  Sum1 : Sum  Inputs=+-
  Sum2 : Sum  Inputs=+-
  Sum29 : Sum
  Sum3 : Sum  Inputs=+-
  Sum31 : Sum
  Sum32 : Sum
  Sum34 : Sum  Inputs=|+-
  Sum35 : Sum  Inputs=+-|
  Sum36 : Sum  Inputs=+++
  Pt_ref : Outport
  Pab_ref : Outport  Port=2
  Pac_ref : Outport  Port=3
  Pula_ref : Outport  Port=4
  Pulb_ref : Outport  Port=5
  Pulc_ref : Outport  Port=6
  wires:
  Product6/1 -> Gain8/1
  Product4/1 -> Gain12/1
  Product2/1 -> Gain10/1
  Product1/1 -> Gain9/1
  Product3/1 -> Gain11/1
  Product5/1 -> Gain7/1
  Sum32/1 -> Sum36/3, Sum35/2
  Sum36/1 -> DC Energy PIs/1(EnergyTotal)
  Sum35/1 -> DC Energy PIs/3(Energydiffac)
  Sum34/1 -> DC Energy PIs/2(Energydiffab)
  Product19/1 -> Gain1/1
  Sum31/1 -> Sum36/2, Sum34/2
  Product17/1 -> Gain6/1
  Sum29/1 -> Sum35/1, Sum34/1, Sum36/1
  Product15/1 -> Gain3/1
  Product14/1 -> Gain2/1
  Product16/1 -> Gain5/1
  Product18/1 -> Gain4/1
  Capvlb/1 -> Product16/2, Product16/1, Product3/2, Product3/1
  Capvub/1 -> Product19/2, Product19/1, Product6/2, Product6/1
  Capvuc/1 -> Product14/2, Product14/1, Product1/2, Product1/1
  Capvua/1 -> Product18/1, Product18/2, Product5/1, Product5/2
  Capvla/1 -> Product15/1, Product15/2, Product2/1, Product2/2
  Capvlc/1 -> Product17/2, Product17/1, Product4/2, Product4/1
  Gain4/1 -> Sum29/1
  Gain1/1 -> Sum31/1
  Gain2/1 -> Sum32/1
  Gain9/1 -> Sum3/1
  Gain8/1 -> Sum2/1
  Gain7/1 -> Sum1/1
  Gain3/1 -> Sum29/2
  Gain5/1 -> Sum31/2
  Gain6/1 -> Sum32/2
  Gain10/1 -> Sum1/2
  Gain12/1 -> Sum3/2
  Gain11/1 -> Sum2/2
  Sum1/1 -> Gain13/1
  Sum2/1 -> Gain14/1
  Sum3/1 -> Gain15/1
  Pt_ffw/1 -> DC Energy PIs/4(ACpowerFFd)
  Pab_ffw/1 -> DC Energy PIs/5(DiffabABpowerFFd)
  Pac_ffw/1 -> DC Energy PIs/6(DiffacACpowerFFd)
  DC Energy PIs/1(TotalPowerRef) -> Pt_ref/1
  DC Energy PIs/3(DiffacPowerRef) -> Pac_ref/1
  DC Energy PIs/2(DiffabPowerRef) -> Pab_ref/1
  AC Power Reference/1(Pdiff_arm_a_Ref) -> Pula_ref/1
  AC Power Reference/2(Pdiff_arm_b_Ref) -> Pulb_ref/1
  AC Power Reference/3(Pdiff_arm_c_Ref) -> Pulc_ref/1
  Gain13/1 -> AC Power Reference/1(Ediff_arm_a)
  Gain15/1 -> AC Power Reference/3(Ediff_arm_c)
  Gain14/1 -> AC Power Reference/2(Ediff_arm_b)

== system MTDC_MODEL/GRID1+MMC1/Equivalent arm lower-a1 ==
  note: Power_la
  vla : Inport
  Controlled Current Source : spsControlledCurrentSourceLib/Controlled Current Source  Initialize=on  Source_Type=AC  Amplitude=0  Phase=0  Frequency=0  Measurements=None
  Controlled Voltage Source7 : spsControlledVoltageSourceLib/Controlled Voltage Source  Initialize=on  Source_Type=AC  Amplitude=Vdc/2  Phase=0  Frequency=0  Measurements=None
  Current Measurement4 : spsCurrentMeasurementLib/Current Measurement  PhasorSimulation=off  OutputType=Complex  PSBequivalent=0
  Divide1 : Product  Inputs=**
  Divide2 : Product  Inputs=*/
  Filtered Lower arm A instananeous power1 : Scope
  Gain : Gain  Gain=1e6
  Lower arm A instananeous power : Scope
  Series RLC Branch2 : spsSeriesRLCBranchLib/Series RLC Branch  LConnTagsString=__new0  RConnTagsString=__new0  BranchType=C  Resistance=Ra_1  Inductance=La_1  SetiL0=on  InitialCurrent=0  Capacitance=Cap/N  Setx0=on  InitialVoltage=640e3  Measurements=None
  Transfer Fcn : TransferFcn  Denominator=[1 1]
  Voltage Measurement : spsVoltageMeasurementLib/Voltage Measurement  PhasorSimulation=off  OutputType=Complex  PSBequivalent=0
  Conn1 : PMIOPort  Side=Right
  Conn2 : PMIOPort  Port=2  Side=Left
  v_sum_la : Outport
  wires:
  Gain/1 -> Filtered Lower arm A instananeous power1/1
  Transfer Fcn/1 -> Gain/1
  Current Measurement4/1 -> Divide1/2  "ila"
  Divide1/1 -> Divide2/1, Transfer Fcn/1, Lower arm A instananeous power/1
  Divide2/1 -> Controlled Current Source/1
  Voltage Measurement/1 -> Divide2/2, v_sum_la/1
  vla/1 -> Controlled Voltage Source7/1, Divide1/1  "vla"
  connections:
  Conn2/RConn1 -- Current Measurement4/RConn1
  Current Measurement4/LConn1 -- Controlled Voltage Source7/LConn1
  Voltage Measurement/LConn2 -- Series RLC Branch2/RConn1 -- Controlled Current Source/LConn1
  Controlled Current Source/RConn1 -- Series RLC Branch2/LConn1 -- Voltage Measurement/LConn1
  Controlled Voltage Source7/RConn1 -- Conn1/RConn1

== system MTDC_MODEL/GRID1+MMC1/Equivalent arm lower-a2 ==
  note: Power_lb
  vlb : Inport
  Controlled Current Source : spsControlledCurrentSourceLib/Controlled Current Source  Initialize=on  Source_Type=AC  Amplitude=0  Phase=0  Frequency=0  Measurements=None
  Controlled Voltage Source7 : spsControlledVoltageSourceLib/Controlled Voltage Source  Initialize=on  Source_Type=AC  Amplitude=Vdc/2  Phase=0  Frequency=0  Measurements=None
  Current Measurement4 : spsCurrentMeasurementLib/Current Measurement  PhasorSimulation=off  OutputType=Complex  PSBequivalent=0
  Divide1 : Product  Inputs=**
  Divide2 : Product  Inputs=*/
  Filtered Lower arm B instananeous power1 : Scope
  Gain : Gain  Gain=1e6
  Lower arm B instananeous power : Scope
  Series RLC Branch2 : spsSeriesRLCBranchLib/Series RLC Branch  LConnTagsString=__new0  RConnTagsString=__new0  BranchType=C  Resistance=Ra_1  Inductance=La_1  SetiL0=on  InitialCurrent=0  Capacitance=Cap/N  Setx0=on  InitialVoltage=640e3  Measurements=None
  Transfer Fcn : TransferFcn  Denominator=[1 1]
  Voltage Measurement : spsVoltageMeasurementLib/Voltage Measurement  PhasorSimulation=off  OutputType=Complex  PSBequivalent=0
  Conn1 : PMIOPort  Side=Right
  Conn2 : PMIOPort  Port=2  Side=Left
  v_sum_lb : Outport
  wires:
  vlb/1 -> Divide1/1, Controlled Voltage Source7/1  "vlb"
  Voltage Measurement/1 -> v_sum_lb/1, Divide2/2
  Divide2/1 -> Controlled Current Source/1
  Divide1/1 -> Lower arm B instananeous power/1, Transfer Fcn/1, Divide2/1
  Current Measurement4/1 -> Divide1/2  "ilb"
  Transfer Fcn/1 -> Gain/1
  Gain/1 -> Filtered Lower arm B instananeous power1/1
  connections:
  Controlled Voltage Source7/RConn1 -- Conn1/RConn1
  Voltage Measurement/LConn1 -- Series RLC Branch2/LConn1 -- Controlled Current Source/RConn1
  Controlled Current Source/LConn1 -- Series RLC Branch2/RConn1 -- Voltage Measurement/LConn2
  Current Measurement4/LConn1 -- Controlled Voltage Source7/LConn1
  Conn2/RConn1 -- Current Measurement4/RConn1

== system MTDC_MODEL/GRID1+MMC1/Equivalent arm lower-a3 ==
  note: Power_lc
  vlc : Inport
  Controlled Current Source : spsControlledCurrentSourceLib/Controlled Current Source  Initialize=on  Source_Type=AC  Amplitude=0  Phase=0  Frequency=0  Measurements=None
  Controlled Voltage Source7 : spsControlledVoltageSourceLib/Controlled Voltage Source  Initialize=on  Source_Type=AC  Amplitude=Vdc/2  Phase=0  Frequency=0  Measurements=None
  Current Measurement4 : spsCurrentMeasurementLib/Current Measurement  PhasorSimulation=off  OutputType=Complex  PSBequivalent=0
  Divide1 : Product  Inputs=**
  Divide2 : Product  Inputs=*/
  Filtered Lower arm A instananeous power1 : Scope
  Gain : Gain  Gain=1e6
  Lower arm A instananeous power : Scope
  Series RLC Branch2 : spsSeriesRLCBranchLib/Series RLC Branch  LConnTagsString=__new0  RConnTagsString=__new0  BranchType=C  Resistance=Ra_1  Inductance=La_1  SetiL0=on  InitialCurrent=0  Capacitance=Cap/N  Setx0=on  InitialVoltage=640e3  Measurements=None
  Transfer Fcn : TransferFcn  Denominator=[1 1]
  Voltage Measurement : spsVoltageMeasurementLib/Voltage Measurement  PhasorSimulation=off  OutputType=Complex  PSBequivalent=0
  Conn1 : PMIOPort  Side=Right
  Conn2 : PMIOPort  Port=2  Side=Left
  v_sum_lc : Outport
  wires:
  Gain/1 -> Filtered Lower arm A instananeous power1/1
  Transfer Fcn/1 -> Gain/1
  Current Measurement4/1 -> Divide1/2  "ila"
  Divide1/1 -> Divide2/1, Transfer Fcn/1, Lower arm A instananeous power/1
  Divide2/1 -> Controlled Current Source/1
  Voltage Measurement/1 -> Divide2/2, v_sum_lc/1
  vlc/1 -> Controlled Voltage Source7/1, Divide1/1  "vla"
  connections:
  Conn2/RConn1 -- Current Measurement4/RConn1
  Current Measurement4/LConn1 -- Controlled Voltage Source7/LConn1
  Voltage Measurement/LConn2 -- Series RLC Branch2/RConn1 -- Controlled Current Source/LConn1
  Controlled Current Source/RConn1 -- Series RLC Branch2/LConn1 -- Voltage Measurement/LConn1
  Controlled Voltage Source7/RConn1 -- Conn1/RConn1

== system MTDC_MODEL/GRID1+MMC1/Equivalent arm upper-a ==
  note: Power_ua
  vua : Inport
  Controlled Current Source : spsControlledCurrentSourceLib/Controlled Current Source  Initialize=on  Source_Type=AC  Amplitude=0  Phase=0  Frequency=0  Measurements=None
  Controlled Voltage Source7 : spsControlledVoltageSourceLib/Controlled Voltage Source  Initialize=on  Source_Type=AC  Amplitude=Vdc/2  Phase=0  Frequency=0  Measurements=None
  Current Measurement4 : spsCurrentMeasurementLib/Current Measurement  PhasorSimulation=off  OutputType=Complex  PSBequivalent=0
  Divide1 : Product  Inputs=**
  Divide2 : Product  Inputs=*/
  Filtered Upper arm A instananeous power1 : Scope
  Gain : Gain  Gain=1e6
  Series RLC Branch2 : spsSeriesRLCBranchLib/Series RLC Branch  LConnTagsString=__new0  RConnTagsString=__new0  BranchType=C  Resistance=Ra_1  Inductance=La_1  SetiL0=on  InitialCurrent=0  Capacitance=Cap/N  Setx0=on  InitialVoltage=640e3  Measurements=None
  Transfer Fcn : TransferFcn  Denominator=[1 1]
  Upper arm A instananeous power : Scope
  Voltage Measurement : spsVoltageMeasurementLib/Voltage Measurement  PhasorSimulation=off  OutputType=Complex  PSBequivalent=0
  Conn1 : PMIOPort  Side=Right
  Conn2 : PMIOPort  Port=2  Side=Left
  v_sum_ua : Outport
  wires:
  vua/1 -> Divide1/1, Controlled Voltage Source7/1  "vua"
  Voltage Measurement/1 -> v_sum_ua/1, Divide2/2
  Divide2/1 -> Controlled Current Source/1
  Divide1/1 -> Upper arm A instananeous power/1, Transfer Fcn/1, Divide2/1
  Current Measurement4/1 -> Divide1/2  "iua"
  Transfer Fcn/1 -> Gain/1
  Gain/1 -> Filtered Upper arm A instananeous power1/1
  connections:
  Controlled Voltage Source7/RConn1 -- Conn1/RConn1
  Voltage Measurement/LConn1 -- Series RLC Branch2/LConn1 -- Controlled Current Source/RConn1
  Controlled Current Source/LConn1 -- Series RLC Branch2/RConn1 -- Voltage Measurement/LConn2
  Current Measurement4/LConn1 -- Controlled Voltage Source7/LConn1
  Conn2/RConn1 -- Current Measurement4/RConn1
